simulink model "Mean_arterial_pressure"  (R2024b)
settings: Solver=VariableStepAuto  StartTime=0.0  StopTime=10.0  RelTol=1e-3
values from neighbouring files (symbols this model uses):
  DBP = input(prompt)    [Mean_arterial_resistance.m]
  PP = input(prompt)    [Mean_arterial_resistance.m]
libraries: simulink x1
settings Model: Creator=Stephon Woodson  LastModifiedBy=Stephon Woodson

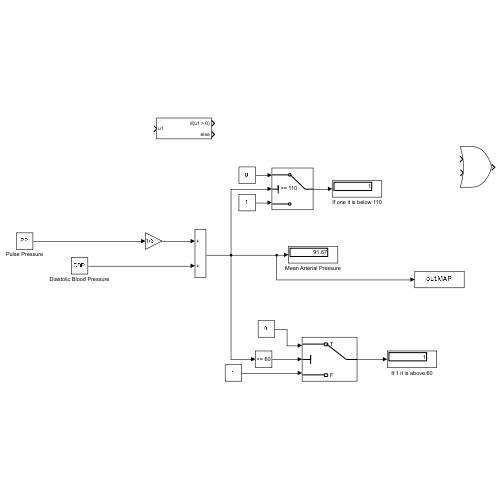
[thumbnail: Simulink's stored preview of the top-level diagram]
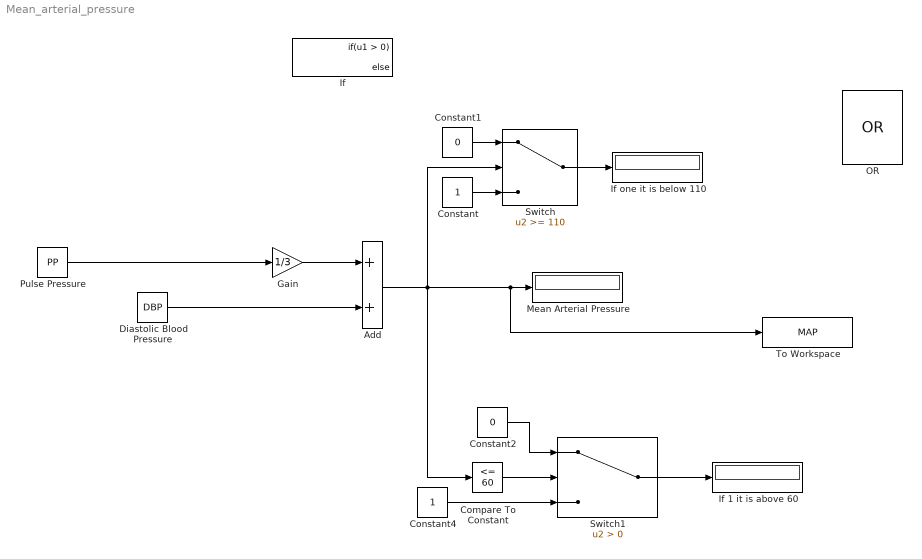
== system Mean_arterial_pressure ==
  Add : Sum
  Compare To Constant : simulink/Logic and Bit Operations/Compare To Constant  relop=<=  const=60  OutDataTypeStr=boolean
  Constant : Constant
  Constant1 : Constant  Value=0
  Constant2 : Constant  Value=0
  Constant4 : Constant
  Diastolic Blood Pressure : Constant  Value=DBP
  Gain : Gain  Gain=1/3
  If : If
  If 1 it is above 60 : Display
  If one it is below 110 : Display
  Mean Arterial Pressure : Display
  OR : Logic  Operator=OR  IconShape=distinctive  AllPortsSameDT=off  OutDataTypeStr=boolean
  Pulse Pressure : Constant  Value=PP
  Switch : Switch  Threshold=110  SaturateOnIntegerOverflow=off  InputSameDT=off
  Switch1 : Switch  Criteria=u2 > Threshold  SaturateOnIntegerOverflow=off  InputSameDT=off
  To Workspace : ToWorkspace  VariableName=MAP  SampleTime=-1
  wires:
  Pulse Pressure/1 -> Gain/1
  Gain/1 -> Add/1
  Diastolic Blood Pressure/1 -> Add/2
  Add/1 -> Compare To Constant/1, Switch/2, To Workspace/1, Mean Arterial Pressure/1
  Constant/1 -> Switch/3
  Constant1/1 -> Switch/1
  Switch/1 -> If one it is below 110/1
  Switch1/1 -> If 1 it is above 60/1
  Compare To Constant/1 -> Switch1/2
  Constant2/1 -> Switch1/1
  Constant4/1 -> Switch1/3
